simulink model "RLC_SIMULATION"  (R2022b)
settings: Solver=VariableStepAuto  StartTime=0.0  StopTime=3e-3  MaxStep=0.000001  RelTol=1e-3
values from neighbouring files (symbols this model uses):
  C = 1e-7    (= 1e-07)    [RLC.m]    (also in RLC_INTEGRACION.m)
  L = 8e-3    (= 0.008)    [RLC.m]    (also in RLC_INTEGRACION.m)
  R = 100    [RLC.m]    (also in RLC_INTEGRACION.m)
libraries: fl_lib x6, nesl_utility x3
settings Model: Creator=Cris  LastModifiedBy=Cris

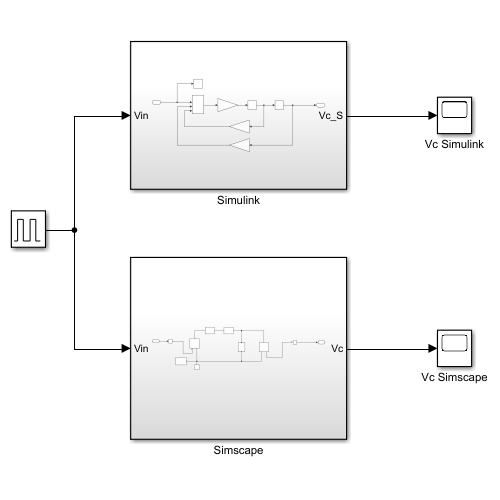
[thumbnail: Simulink's stored preview of the top-level diagram]
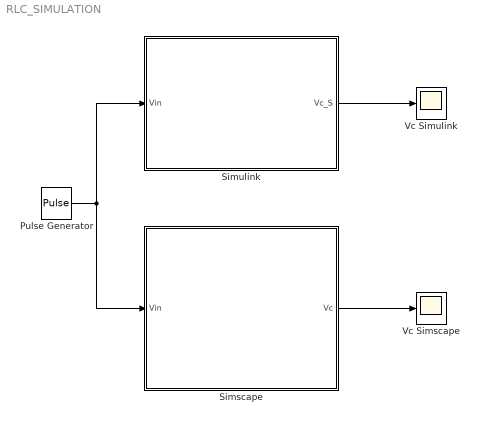
== system RLC_SIMULATION ==
  Pulse Generator : DiscretePulseGenerator  PulseType=Time based  Amplitude=5  Period=0.002  PulseWidth=50
  Simscape : Subsystem
  Simulink : Subsystem
  Vc Simscape : Scope
  Vc Simulink : Scope
  wires:
  Pulse Generator/1 -> Simulink/1(Vin), Simscape/1(Vin)
  Simulink/1(Vc_S) -> Vc Simulink/1
  Simscape/1(Vc) -> Vc Simscape/1

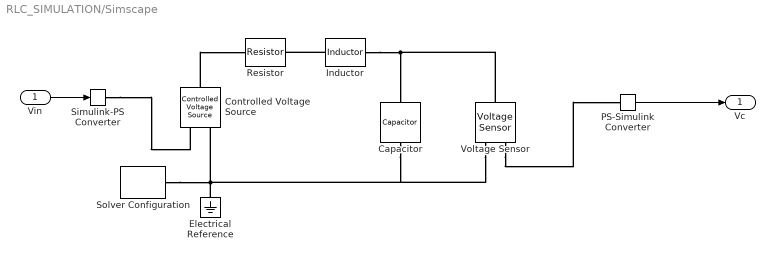
== system RLC_SIMULATION/Simscape ==
  Vin : Inport
  Capacitor : fl_lib/Electrical/Electrical Elements/Capacitor  c=C F  r=1e-6 Ohm  g=0 1/Ohm  i_specify=off  i_priority=None  i=0 A  i_nominal_specify=off  i_nominal_unit=A  i_nominal_value=1  v_specify=off  v_priority=None  v=0 V  v_nominal_specify=off  v_nominal_unit=V  v_nominal_value=1  vc_specify=off  vc_priority=High  vc=0 V  vc_nominal_specify=off  vc_nominal_unit=V  vc_nominal_value=1
  Controlled Voltage Source : fl_lib/Electrical/Electrical Sources/Controlled Voltage Source
  Electrical Reference : fl_lib/Electrical/Electrical Elements/Electrical Reference
  Inductor : fl_lib/Electrical/Electrical Elements/Inductor  l=L H  r=0 Ohm  g=1e-9 1/Ohm  i_specify=off  i_priority=None  i=0 A  i_nominal_specify=off  i_nominal_unit=A  i_nominal_value=1  v_specify=off  v_priority=None  v=0 V  v_nominal_specify=off  v_nominal_unit=V  v_nominal_value=1  i_L_specify=off  i_L_priority=High  i_L=0 A  i_L_nominal_specify=off  i_L_nominal_unit=A  i_L_nominal_value=1
  PS-Simulink Converter : nesl_utility/PS-Simulink Converter  PhysicalDomain=network_engine_domain  SubClassName=ps_output  LeftPortType=input  RightPortType=output  PseudoPeriodic=off  Frequencies=[]  VectorFormat=inherit  Unit=inherit  AffineConversion=off
  Resistor : fl_lib/Electrical/Electrical Elements/Resistor  R=R Ohm  i_specify=off  i_priority=None  i=0 A  i_nominal_specify=off  i_nominal_unit=A  i_nominal_value=1  v_specify=off  v_priority=None  v=0 V  v_nominal_specify=off  v_nominal_unit=V  v_nominal_value=1
  Simulink-PS Converter : nesl_utility/Simulink-PS Converter  PhysicalDomain=network_engine_domain  SubClassName=ps_input  LeftPortType=input  RightPortType=output  PseudoPeriodic=off  Frequencies=[]  NoiseDistribution=none  NoiseParameters=[]  Unit=1  AffineConversion=off  FilteringAndDerivatives=provide  SimscapeFilterOrder=1  InputFilterTimeConstant=0.001  UdotUserProvided=0
  Solver Configuration : nesl_utility/Solver Configuration  PhysicalDomain=network_engine_domain  SubClassName=solver  LeftPortType=input  RightPortType=generic  Tones=[]  Harmonics=[]  SimulateNoise=off  Profile=off  UseLocalSampling=off  EnableSwitchedLinearOptims=on  FrequencyDomain=off  UseCCode=off  RelTol=0.001  AbsTol=0.001  MinStep=1e-09  ToWorkspace=off  RevertToSquareIcSolve=off  NumHomotopyIterations=100  PhasorMode=off  PhasorModeNumHarmonics=1  ConsistencySolver=NEWTON_XTOL_AFTER_FTOL  IndexReductionMethod=DerivativeReplacement  DoDC=off  ResidualTolerance=1e-09  ConsistencyTolSource=GLOBAL  ConsistencyAbsTol=0.001  ConsistencyRelTol=0.001  ConsistencyTolFactor=0.001  UseLocalSolver=off  LocalSolverChoice=NE_BACKWARD_EULER_ADVANCER  ResolveIndetEquations=on  FunctionEvalNumThread=1  LocalSolverSampleTime=0.001  DoFixedCost=off  MaxNonlinIter=3  MaxModeIter=2  ComputeImpulses=off  ImpulseIterations=2  LinearAlgebra=auto  LinearAlgebraNumThread=0  EquationFormulation=NE_TIME_EF  DelaysMemoryBudget=1024  AutomaticFiltering=on  FilteringTimeConstant=0.001  PartitionStorageMethod=AS_NEEDED  PartitionMemoryBudget=1024  PartitionMethod=ROBUST
  Voltage Sensor : fl_lib/Electrical/Electrical Sensors/Voltage Sensor
  Vc : Outport
  wires:
  PS-Simulink Converter/1 -> Vc/1
  Vin/1 -> Simulink-PS Converter/1
  connections:
  Electrical Reference/LConn1 -- Capacitor/RConn1 -- Voltage Sensor/RConn2 -- Controlled Voltage Source/RConn2 -- Solver Configuration/RConn1
  Simulink-PS Converter/RConn1 -- Controlled Voltage Source/RConn1
  Controlled Voltage Source/LConn1 -- Resistor/LConn1
  Voltage Sensor/RConn1 -- PS-Simulink Converter/LConn1
  Inductor/LConn1 -- Resistor/RConn1
  Inductor/RConn1 -- Voltage Sensor/LConn1 -- Capacitor/LConn1

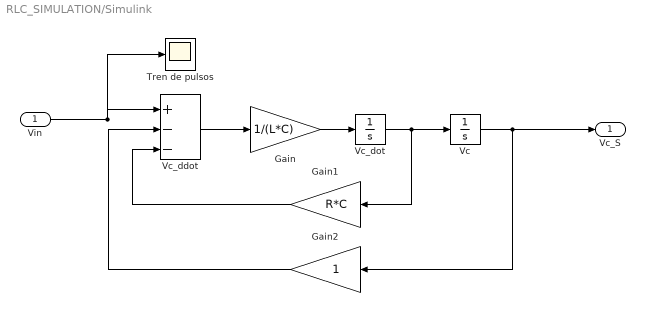
== system RLC_SIMULATION/Simulink ==
  Vin : Inport
  Gain : Gain  Gain=1/(L*C)
  Gain1 : Gain  Gain=R*C
  Gain2 : Gain
  Tren de pulsos : Scope
  Vc : Integrator
  Vc_ddot : Sum  Inputs=|+--
  Vc_dot : Integrator
  Vc_S : Outport
  wires:
  Vc_dot/1 -> Gain1/1, Vc/1
  Gain/1 -> Vc_dot/1
  Vin/1 -> Tren de pulsos/1, Vc_ddot/1
  Vc_ddot/1 -> Gain/1
  Gain1/1 -> Vc_ddot/3
  Gain2/1 -> Vc_ddot/2
  Vc/1 -> Vc_S/1, Gain2/1
